simulink model "power_HEV_powertrain"  (Simulink 8.5)
settings: Solver=ode23tb  StartTime=0.0  StopTime=16  MaxStep=Ts  RelTol=1e-3
InitFcn:
  | Pbatt = 21e3;
  | Vbatt = 100;
  | 
  | Ts = 6e-5;   % time step
  | Kb = -2.6;     % planetary gear ratio
  | 
  | MotorNomSpeed = 1200; %rpm
  | MotorMaxTorque = 400; % Nm
  | AccelGain = 1.1;
undefined symbols (not defined in the file): Hydride, magnitude, Metal, Nickel, speed
libraries: powerlib x47, driveline x32, simulink x11, simulink_extras x9, powerlib_extras x4, electricdrivelib x3, DC6DriveInternalModels x1
(part 1 of 3)
Description:
  | Copyright 2008-2011 The MathWorks, Inc.
CloseFcn:
  | rtwprivate ssgensfun ModelCloseRequest power_HEV_powertrain
settings Model: Creator=MathWorks  LastModifiedBy=Elena  CovSFcnEnable=off  ExtModeAutoUpdateStatusClock=off
settings OptimizationCC: OptimizeBlockIOStorage=off  BufferReuse=off  GlobalBufferReuse=off  ExpressionFolding=off  LocalBlockOutputs=off  InitFltsAndDblsToZero=on
settings DebuggingCC: SignalResolutionControl=TryResolveAllWithWarning  SolverPrmCheckMsg=warning  MultiTaskDSMMsg=warning  MultiTaskCondExecSysMsg=none  SigSpecEnsureSampleTimeMsg=none  FcnCallInpInsideContextMsg=UseLocalSettings  UnknownTsInhSupMsg=none
settings HardwareCC: TargetEndianess=LittleEndian  TargetHWDeviceType=MATLAB Host  ProdEqTarget=off

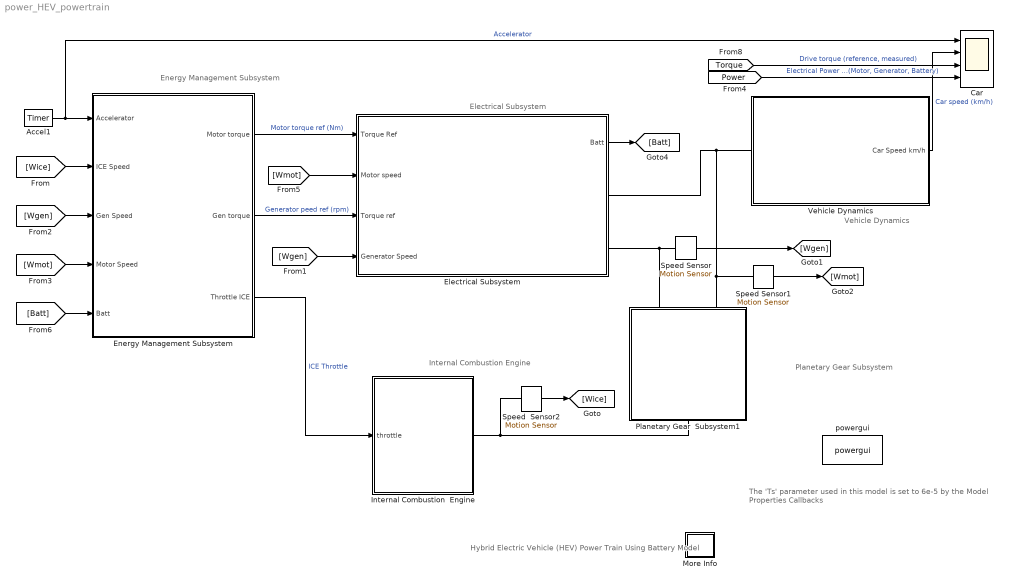
== system power_HEV_powertrain ==
  note: The 'Ts' parameter used in this model
      | is set to 6e-5  by the Model Properties Callbacks
  note: Energy Management
      | Subsystem
  note: Internal Combustion
      | Engine
  note: Planetary Gear
      | Subsystem
  note: Vehicle Dynamics
  note: Hybrid Electric Vehicle (HEV) Power Train Using Battery Model
  note: Electrical Subsystem
  Accel1 : powerlib_extras/Control  Blocks/Timer  t=[0 4 8 13]  e=[0.7 0.1 0.85 -0.7]
  Car : Scope  NumInputPorts=4
      settings: TimeRange=16  YMin=-0.7~-5~-250~-25000  YMax=0.9~75~350~50000  SaveName=ScopeData3  Decimation=10
  Electrical Subsystem : Subsystem
      mask Display: image(imread('power_HEV_powertrain_electrical2.png'))
  Energy Management Subsystem : Subsystem
      mask init:
      | [X1,X1m,X2,X2m,X3,X4,Y1,Y1m,Y2,Y2m,Y3,Y4,color1,color2]=spsdrivelogo;
      | power_max = 57000;
      | speed_at_power_max = 5000;
      | speed_max = 6000;
      | [speed,power,torque,p] = drive_enginemodel('MaskGasoline');
      mask Display:
      | patch([X1 X1m],[Y1 Y1m],color1);
      | patch(X3,Y3,color2);
      | plot([X1 X1m X2 X2m X3 X4],[Y1 Y1m Y2 Y2m Y3 Y4]);
  Internal Combustion  Engine : Subsystem
      mask Display: image(imread('power_HEV_powertrain_THS.jpg'))
  More Info : Subsystem
      settings: OpenFcn=showdemo('power_HEV_powertrain');
      mask Display: disp('?')
  Planetary Gear  Subsystem1 : Subsystem
      mask Display: image(imread('power_HEV_powertrain_planetary2.jpg'));
  Speed Sensor : driveline/Sensors & Actuators/Motion Sensor  Angle=off  x0=0  Velocity=on  Acceleration=off
  Speed Sensor1 : driveline/Sensors & Actuators/Motion Sensor  Angle=off  x0=0  Velocity=on  Acceleration=off
  Speed  Sensor2 : driveline/Sensors & Actuators/Motion Sensor  Angle=off  x0=0  Velocity=on  Acceleration=off
  Vehicle Dynamics : Subsystem
      mask Display: image(imread('power_powertrain_car.jpg'))
  powergui : powerlib/powergui  SimulationMode=Discrete  SolverType=Tustin  SampleTime=6e-5  frequency=60  SPID=off  DisableSnubberDevices=off  DisableRonSwitches=off  DisableVfSwitches=off  SwTol=0  DisplayEquations=off  Interpol=off  methode=off  Ts=0  FunctionMessages=off  echomessages=off  HookPort=off  EnableUseOfTLC=off  x0status=blocks  frequencyindice=0  Pbase=100e6  ErrMax=1e-4  Iterations=50  UnitsV=kV  UnitsW=MW  buscounter=0  RestoreLinks=warning  ResistiveCurrentMeasurement=off  Frange=[0:2:500]  Ylog=off  Xlog=on  ShowGrid=off  save=off  variable=ZData  structure=0  ZoomFFT=on  StartTime=0.0  cycles=1  DisplayStyle=1  fundamental=60  FreqAxis=off  MaxFrequency=1000  frequencyindicesteady=1  RmsSteady=1  display=off
  wires:
  Energy Management Subsystem/1(Motor torque) -> Electrical Subsystem/1(Torque Ref)  "Motor torque ref (Nm)"
  Energy Management Subsystem/2(Gen torque) -> Electrical Subsystem/3(Torque ref)  "Generator peed ref (rpm)"
  Accel1/1 -> Energy Management Subsystem/1(Accelerator), Car/1  "Accelerator"
  Speed Sensor/1 -> [Wgen]
  [Wgen] -> Electrical Subsystem/4(Generator Speed)
  [Wgen] -> Energy Management Subsystem/3(Gen Speed)
  Speed Sensor1/1 -> [Wmot]
  [Wmot] -> Energy Management Subsystem/4(Motor Speed)
  [Wmot] -> Electrical Subsystem/2(Motor speed)
  [Wice] -> Energy Management Subsystem/2(ICE Speed)
  Electrical Subsystem/1(Batt) -> [Batt]
  [Batt] -> Energy Management Subsystem/5(Batt)
  Energy Management Subsystem/3(Throttle ICE) -> Internal Combustion  Engine/1(throttle)  "ICE Throttle"
  Speed  Sensor2/1 -> [Wice]
  [Power] -> Car/4  "Electrical Power (Motor, Generator, Battery)"
  [Torque] -> Car/3  "Drive torque (reference, measured)"
  Vehicle Dynamics/1(Car Speed km/h) -> Car/2  "Car speed (km/h)"
  connections:
  Electrical Subsystem/RConn2 -- Planetary Gear  Subsystem1/RConn1 -- Speed Sensor/LConn1
  Internal Combustion  Engine/RConn1 -- Planetary Gear  Subsystem1/LConn1 -- Speed  Sensor2/LConn1
  Planetary Gear  Subsystem1/RConn2 -- Electrical Subsystem/RConn1 -- Vehicle Dynamics/LConn1 -- Speed Sensor1/LConn1

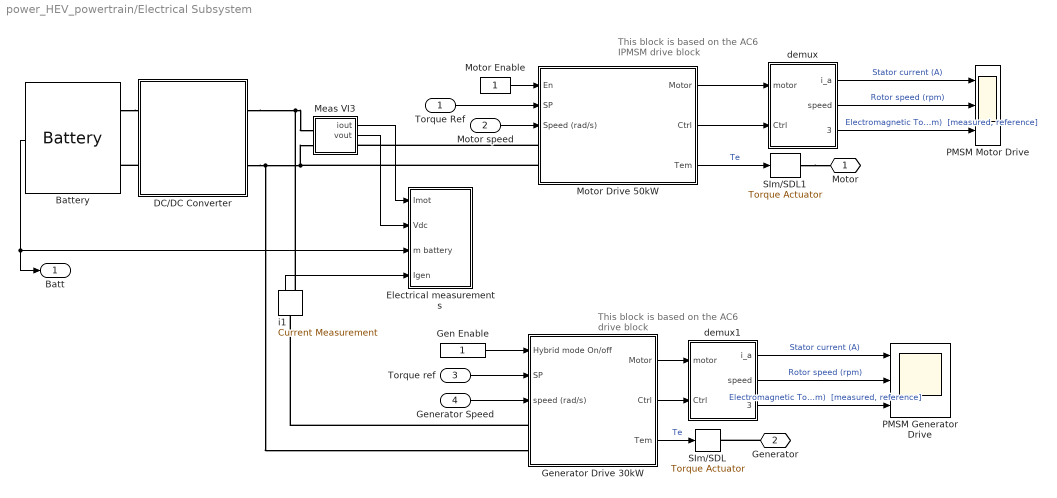
== system power_HEV_powertrain/Electrical Subsystem ==
  note: This block is based on the
      | AC6 IPMSM drive block
  note: This block is based on the AC6
      | drive block
  Torque Ref : Inport
  Motor speed : Inport  Port=2
  Torque ref : Inport  Port=3
  Generator Speed : Inport  Port=4
  Battery : electricdrivelib/Extra Sources/Battery  BatType=Nickel-Metal-Hydride  ShowDetailedParameters=off  NomV=200  NomQ=6.5  SOC=41.53  PresetModel=on  MaxQ=7  FullV=235.5932  Dis_rate=1.3  R=0.30769  Normal_OP=6.25  expZone="[216.9492           1.3]"  current=[50 100]  Units=Time  Batt_Tr=30
  DC/DC Converter : Subsystem
      mask init:
      | [X1,X1m,X2,X2m,X3,X4,Y1,Y1m,Y2,Y2m,Y3,Y4,color1,color2]=spsdrivelogo;
      mask Display:
      | patch([X1 X1m],[Y1 Y1m],color1);
      | patch(X3,Y3,color2);
      | plot([X1 X1m X2 X2m X3 X4],[Y1 Y1m Y2 Y2m Y3 Y4]);
  Electrical measurements : Subsystem
  Gen Enable : Constant
  Generator Drive 30kW : Subsystem
      mask Display: image(imread('power_HEV_powertrain_syncgenerator.jpg'))
  Meas VI3 : Subsystem
  Motor Drive 50kW : Subsystem
      mask Display: image(imread('power_HEV_powertrain_syncmotor.jpg'))
  Motor Enable : Constant
  PMSM Generator Drive : Scope  NumInputPorts=3
      settings: TimeRange=16  YMin=-150~-2000~-35  YMax=150~14000~5  SaveName=simout2  Decimation=10
  PMSM Motor Drive : Scope  NumInputPorts=3
      settings: TimeRange=16  YMin=-250~0~-100  YMax=250~3500~300  SaveName=simout5  Decimation=10
  SIm/SDL : driveline/Sensors & Actuators/Torque Actuator
  SIm/SDL1 : driveline/Sensors & Actuators/Torque Actuator
  demux : Subsystem
  demux1 : Subsystem
  i1 : powerlib/Measurements/Current Measurement  PhasorSimulation=off  OutputType=Complex  PSBequivalent=0
  Motor : PMIOPort  Port=1  Side=Right
  Generator : PMIOPort  Port=2  Side=Right
  Batt : Outport
  wires:
  i1/1 -> Electrical measurements/4(Igen)
  Meas VI3/2(vout) -> Electrical measurements/2(Vdc)
  Meas VI3/1(iout) -> Electrical measurements/1(Imot)
  Torque ref/1 -> Generator Drive 30kW/2(SP)
  Generator Speed/1 -> Generator Drive 30kW/3(speed (rad/s))
  Gen Enable/1 -> Generator Drive 30kW/1(Hybrid mode On/off)
  Battery/1 -> Electrical measurements/3(m battery), Batt/1
  Generator Drive 30kW/3(Tem) -> SIm/SDL/1  "Te"
  demux1/2(speed) -> PMSM Generator Drive/2  "Rotor speed (rpm)"
  demux1/3(Torque) -> PMSM Generator Drive/3  "Electromagnetic Torque (Nm)  [measured, reference]"
  demux1/1(i_a) -> PMSM Generator Drive/1  "Stator current (A)"
  Generator Drive 30kW/1(Motor) -> demux1/1(motor)
  Generator Drive 30kW/2(Ctrl) -> demux1/2(Ctrl)
  Motor Enable/1 -> Motor Drive 50kW/1(En)
  Motor speed/1 -> Motor Drive 50kW/3(Speed (rad/s))
  Torque Ref/1 -> Motor Drive 50kW/2(SP)
  Motor Drive 50kW/3(Tem) -> SIm/SDL1/1  "Te"
  Motor Drive 50kW/1(Motor) -> demux/1(motor)
  Motor Drive 50kW/2(Ctrl) -> demux/2(Ctrl)
  demux/2(speed) -> PMSM Motor Drive/2  "Rotor speed (rpm)"
  demux/3(Torque) -> PMSM Motor Drive/3  "Electromagnetic Torque (Nm)  [measured, reference]"
  demux/1(i_a) -> PMSM Motor Drive/1  "Stator current (A)"
  connections:
  DC/DC Converter/LConn2 -- Battery/LConn2
  Battery/LConn1 -- DC/DC Converter/LConn1
  Generator/RConn1 -- SIm/SDL/RConn1
  Motor Drive 50kW/LConn1 -- Meas VI3/RConn1
  DC/DC Converter/RConn1 -- Meas VI3/LConn1 -- i1/RConn1
  Generator Drive 30kW/LConn1 -- i1/LConn1
  DC/DC Converter/RConn2 -- Generator Drive 30kW/LConn2 -- Motor Drive 50kW/LConn2 -- Meas VI3/LConn2
  SIm/SDL1/RConn1 -- Motor/RConn1

== system power_HEV_powertrain/Energy Management Subsystem ==
  Accelerator : Inport
  ICE Speed : Inport  Port=2
  Gen Speed : Inport  Port=3
  Motor Speed : Inport  Port=4
  Batt : Inport  Port=5
  " 2" : Gain  Gain=-1
  Battery Management System : Subsystem
      mask init:
      | [X1,X1m,X2,X2m,X3,X4,Y1,Y1m,Y2,Y2m,Y3,Y4,color1,color2]=spsdrivelogo;
      mask Display:
      | patch([X1 X1m],[Y1 Y1m],color1);
      | patch(X3,Y3,color2);
      | plot([X1 X1m X2 X2m X3 X4],[Y1 Y1m Y2 Y2m Y3 Y4]);
  Drive torque1 : Product  Inputs=**  OutDataTypeStr=double
  Hybrid Management System : Subsystem
      mask init:
      | [X1,X1m,X2,X2m,X3,X4,Y1,Y1m,Y2,Y2m,Y3,Y4,color1,color2]=spsdrivelogo;
      mask Display:
      | patch([X1 X1m],[Y1 Y1m],color1);
      | patch(X3,Y3,color2);
      | plot([X1 X1m X2 X2m X3 X4],[Y1 Y1m Y2 Y2m Y3 Y4]);
  ICE Speed Controller : Subsystem  mask(Speed controller){SwK=Speed regulation, bs=1800, ramp=[-5000,5000]*10, kp=0.01, ki=0.1, fc=100, ctrl_sat=[0,1], Tsc=Ts}
      mask prompts: SwK "Regulation type"; bs "Base speed (rpm)"; ramp "Speed reference ramp (rpm/s) [deceleration,acceleration]"; kp "Proportional gain"; ki "Integral gain"; fc "Speed measurement - low-pass filter cutoff frequency (Hz)"; ctrl_sat "Controller output torque saturation (N.m) [negative,positive]"; Tsc "Controller sampling time (s)"
      mask help: This block implements a PI speed regulator.
      mask init:
      | [X1,X1m,X2,X2m,X3,X4,Y1,Y1m,Y2,Y2m,Y3,Y4,color1,color2]=spsdrivelogo;
      mask TypeOptions SwK: Speed regulation | Torque regulation
      mask Display:
      | patch([X1 X1m],[Y1 Y1m],color1);
      | patch(X3,Y3,color2);
      | plot([X1 X1m X2 X2m X3 X4],[Y1 Y1m Y2 Y2m Y3 Y4]);
  Rate Limiter : RateLimiter  RisingSlewLimit=10  FallingSlewLimit=-10  SampleTimeMode=inherited
  Scope2 : Scope  NumInputPorts=2
      settings: TimeRange=10  YMin=0~0  YMax=525~7500  SaveName=ScopeData13  Decimation=10
  Terminator : Terminator
  Torque limitation : Subsystem
      mask Display: plot([0;1800;2000;2500;3000;3500], [1;1;0.90*1;0.72*1;0.6*1;0.51*1])
  Motor torque : Outport
  Gen torque : Outport  Port=2
  Throttle ICE : Outport  Port=3
  wires:
  Gen Speed/1 -> Hybrid Management System/6(Generator speed (rad/s))  "Generator speed (rad/s)"
  Motor Speed/1 -> Hybrid Management System/5(Motor speed (rad/s)), Drive torque1/2, Torque limitation/2(N rad/s)  "Motor speed (rad/s)"
  Batt/1 -> Battery Management System/1(Batt)
  Accelerator/1 -> Rate Limiter/1
  ICE Speed/1 -> Hybrid Management System/7(ICE speed (rad/s)), ICE Speed Controller/3(N)
  Hybrid Management System/3(Hybrid Enable) -> ICE Speed Controller/1(En)
  Hybrid Management System/1(Motor torque ref) -> Motor torque/1
  Hybrid Management System/2(Gen torque ref) -> " 2"/1
  ICE Speed Controller/1(Torque*) -> Throttle ICE/1
  ICE Speed Controller/2(Ctrl) -> Terminator/1
  Torque limitation/1(torque) -> Drive torque1/1, Hybrid Management System/3(Drive torque), Scope2/1  "Required torque"
  Drive torque1/1 -> Scope2/2, Hybrid Management System/4(Drive power)  "Required drive power"
  Hybrid Management System/4(ICE speed ref (rpm)) -> ICE Speed Controller/2(N*)
  Battery Management System/1(Battery power) -> Hybrid Management System/1(Recharge power)
  Battery Management System/2(Battery limit) -> Hybrid Management System/2(Battery Limit)
  Rate Limiter/1 -> Torque limitation/1(Torque)
  " 2"/1 -> Gen torque/1

== system power_HEV_powertrain/Internal Combustion  Engine ==
  throttle : Inport
  Driveline Environment : driveline/Solver & Inertias/Driveline Environment  PortType=p1  BlockClass=Solver  PhysicalDomain=driveline_domain  SimulationMode=Dynamics  ModeIteration=off  DefaultClutchVelocityTolerance=1e-3  DefaultUseAutoClutchVelocityTolerance=on
  Gasoline Engine : driveline/Vehicle Components/Gasoline Engine  power_max=57000+57000  speed_at_power_max=5000  speed_max=6000
  Housing : driveline/Solver & Inertias/Housing
  ICE : Scope  NumInputPorts=4
      settings: TimeRange=16  YMin=0~0~-10~-5000  YMax=1~5500~130~50000  SaveName=ScopeData7  Decimation=10
  ICE friction 57 kW @ 5000 rpm : driveline/Dynamic Elements/Torsional  Spring-Damper  k=0  c=0.2079  x0=0  Backlash=0
  Inertia : driveline/Solver & Inertias/Inertia  PortType=p1  BlockClass=Inertia  PhysicalDomain=driveline_domain  I=0.25  Ip=[]  Iv=[]  ShowLeft=off  ShowRight=on
  Motion Sensor : driveline/Sensors & Actuators/Motion Sensor  Angle=off  x0=0  Velocity=on  Acceleration=off
  Product : Product  RndMeth=Zero
  Product1 : Product  RndMeth=Zero
  T1 : driveline/Sensors & Actuators/Torque Sensor
  rad/s to rpm : Constant  Value=60/(2*pi)
  Engine : PMIOPort  Port=1  Side=Right
  tag scope: T_ICE=global
  wires:
  rad/s to rpm/1 -> Product/2
  Motion Sensor/1 -> Product/1, Product1/1
  throttle/1 -> ICE/1, Gasoline Engine/1  "Throttle"
  Product/1 -> ICE/2  "Engine speed (rpm)"
  Product1/1 -> ICE/4  "engine power (w)"
  T1/1 -> Product1/2, [T_ICE], ICE/3  "engine torque (Nm)"
  connections:
  ICE friction 57 kW @ 5000 rpm/LConn1 -- T1/LConn1 -- Inertia/RConn1 -- Motion Sensor/LConn1 -- Gasoline Engine/RConn1 -- Driveline Environment/LConn1
  T1/RConn1 -- Engine/RConn1
  Housing/RConn1 -- ICE friction 57 kW @ 5000 rpm/RConn1

== system power_HEV_powertrain/More Info ==

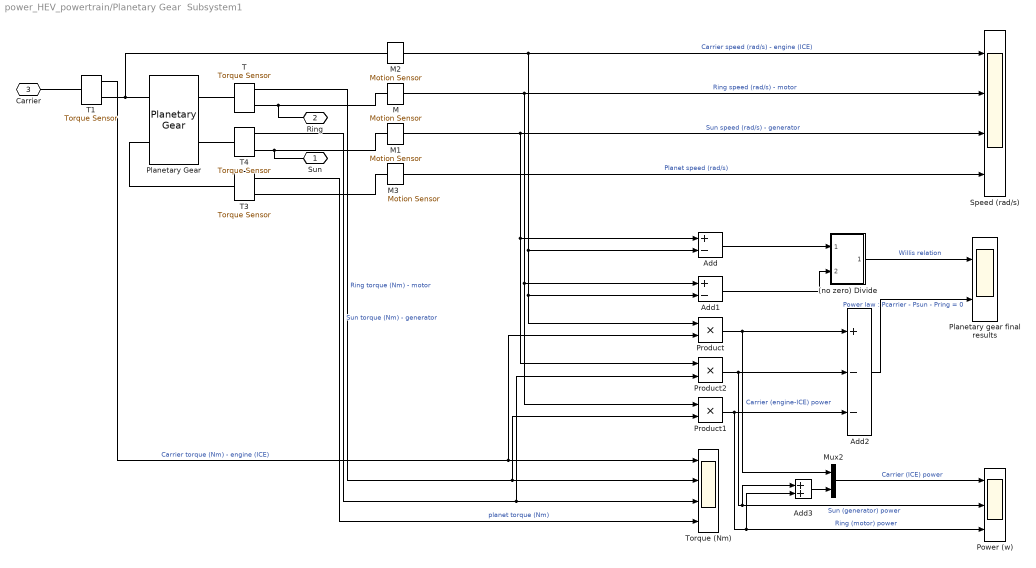
== system power_HEV_powertrain/Planetary Gear  Subsystem1 ==
  (no zero) Divide : Subsystem
  Add : Sum  Inputs=+-
  Add1 : Sum  Inputs=+-
  Add2 : Sum  Inputs=+--
  Add3 : Sum
  M{,1..3} (4 alike) : driveline/Sensors & Actuators/Motion Sensor  Angle=off  x0=0  Velocity=on  Acceleration=off
  Mux2 : Mux  Inputs=2
  Planetary Gear : driveline/Gears/Planetary Gear  Ratio=-Kb  Show=on  LinearizationFlag=off  ValidatorFcn=drive_planetarygearblock
  Planetary gear final results : Scope  NumInputPorts=2
      settings: TimeRange=16  YMin=-3~-1e-010  YMax=0~3e-010  Decimation=10
  Power (w) : Scope  NumInputPorts=3
      settings: TimeRange=16  YMin=-10000~-10000~-2000  YMax=60000~50000~12000  Decimation=10
  Product : Product  RndMeth=Zero
  Product1 : Product  RndMeth=Zero
  Product2 : Product  RndMeth=Zero
  Speed (rad/s) : Scope  NumInputPorts=4
      settings: TimeRange=16  YMin=-100~-20~-200~-400  YMax=500~120~1200~100  SaveName=ScopeData2  Decimation=10
  T{,1,3..4} (4 alike) : driveline/Sensors & Actuators/Torque Sensor
  Torque (Nm) : Scope  NumInputPorts=4
      settings: TimeRange=16  YMin=-50~-20~-10~-2e-013  YMax=150~100~40~6.000000000000001e-013  SaveName=ScopeData4  Decimation=10
  Sun : PMIOPort  Port=1  Side=Right
  Ring : PMIOPort  Port=2  Side=Right
  Carrier : PMIOPort  Port=3  Side=Left
  wires:
  M/1 -> Add1/1, Product1/1, Speed (rad/s)/2  "Ring speed (rad/s) - motor"
  M1/1 -> Speed (rad/s)/3, Add/1, Product2/1  "Sun speed (rad/s) - generator"
  T/1 -> Torque (Nm)/2, Product1/2  "Ring torque (Nm) - motor"
  M2/1 -> Speed (rad/s)/1, Add/2, Add1/2, Product/1  "Carrier speed (rad/s) - engine (ICE)"
  M3/1 -> Speed (rad/s)/4  "Planet speed (rad/s)"
  T3/1 -> Torque (Nm)/4  "planet torque (Nm)"
  T4/1 -> Torque (Nm)/3, Product2/2  "Sun torque (Nm) - generator"
  Add1/1 -> (no zero) Divide/2(SP2)
  (no zero) Divide/1(WR) -> Planetary gear final results/1  "Willis relation"
  Product/1 -> Add2/1, Mux2/1  "Carrier (engine-ICE) power"
  Product2/1 -> Add2/2, Power (w)/2, Add3/1  "Sun (generator) power"
  Product1/1 -> Add2/3, Power (w)/3, Add3/2  "Ring (motor) power"
  Add2/1 -> Planetary gear final results/2  "Power law : Pcarrier - Psun - Pring = 0"
  T1/1 -> Torque (Nm)/1, Product/2  "Carrier torque (Nm) - engine (ICE)"
  Add3/1 -> Mux2/2
  Mux2/1 -> Power (w)/1  "Carrier (ICE) power"
  Add/1 -> (no zero) Divide/1(SP1)
  connections:
  Planetary Gear/LConn1 -- M2/LConn1 -- T1/RConn1
  M1/LConn1 -- T4/RConn1 -- Sun/RConn1
  Planetary Gear/RConn1 -- T/LConn1
  Planetary Gear/RConn2 -- T4/LConn1
  T3/LConn1 -- Planetary Gear/LConn2
  M/LConn1 -- T/RConn1 -- Ring/RConn1
  T3/RConn1 -- M3/LConn1
  T1/LConn1 -- Carrier/RConn1

== system power_HEV_powertrain/Vehicle Dynamics ==
  Differential : driveline/Gears/Differential  R=1  ValidatorFcn=drive_differentialgearblock  SimDrivelineLibraryVersion=1.1
  Housing : driveline/Solver & Inertias/Housing
  Longitudinal Vehicle Dynamics : driveline/Vehicle Components/Longitudinal Vehicle Dynamics  m=1325  a=1.35  b=1.35  h=0.5  FA=2.57  C_d=0.26  v0=0
  Simple Gear : driveline/Gears/Simple Gear  PortType=p1  BlockClass=SimpleGear  PhysicalDomain=driveline_domain  Reversing=off  Ratio=4.113
  Terminator : Terminator
  Terminator1 : Terminator
  Tire : driveline/Vehicle Components/Tire  r_e=0.3  F_z=3000  F_x_max=3500  kappa_max=10  sigma_k=0.2
  Tire1 : driveline/Vehicle Components/Tire  r_e=0.3  F_z=3000  F_x_max=3500  kappa_max=10  sigma_k=0.2
  Torque after gear1 : driveline/Sensors & Actuators/Torque Sensor
  Total friction : driveline/Dynamic Elements/Torsional  Spring-Damper  k=0  c=0.1  x0=0  Backlash=0
  Transmision inertia : driveline/Solver & Inertias/Inertia  PortType=p1  BlockClass=Inertia  PhysicalDomain=driveline_domain  I=0.5  Ip=[]  Iv=[]  ShowLeft=off  ShowRight=on
  m/s to km/h : Gain  Gain=(60*60)/1000
  road angle : Constant  Value=0
  tire inertia : driveline/Solver & Inertias/Inertia  PortType=p1  BlockClass=Inertia  PhysicalDomain=driveline_domain  I=0.5  Ip=[]  Iv=[]  ShowLeft=off  ShowRight=on
  tire inertia1 : driveline/Solver & Inertias/Inertia  PortType=p1  BlockClass=Inertia  PhysicalDomain=driveline_domain  I=0.5  Ip=[]  Iv=[]  ShowLeft=off  ShowRight=on
  Drive Shaft : PMIOPort  Port=1  Side=Left
  Car Speed km/h : Outport
  tag scope: DriveTorque=global
  wires:
  road angle/1 -> Longitudinal Vehicle Dynamics/3
  Tire1/2 -> Longitudinal Vehicle Dynamics/1
  Tire/2 -> Longitudinal Vehicle Dynamics/2
  Tire1/1 -> Terminator/1
  Tire/1 -> Terminator1/1
  Longitudinal Vehicle Dynamics/1 -> Tire/1, Tire1/1, m/s to km/h/1
  Longitudinal Vehicle Dynamics/2 -> Tire1/2
  Longitudinal Vehicle Dynamics/3 -> Tire/2
  m/s to km/h/1 -> Car Speed km/h/1
  Torque after gear1/1 -> [DriveTorque]  "Drive shaft torque"
  connections:
  Differential/RConn1 -- Tire1/LConn1 -- tire inertia1/RConn1
  Differential/RConn2 -- Tire/LConn1 -- tire inertia/RConn1
  Drive Shaft/RConn1 -- Torque after gear1/LConn1
  Torque after gear1/RConn1 -- Simple Gear/LConn1 -- Total friction/RConn1
  Differential/LConn1 -- Simple Gear/RConn1 -- Transmision inertia/RConn1
  Housing/RConn1 -- Total friction/LConn1

== system power_HEV_powertrain/Electrical Subsystem/DC/DC Converter ==
  Bus DC controller : Subsystem
  DC/DC converter : Subsystem
  Ubus Ref : Constant  Value=500
  +Vdc Bus : PMIOPort  Tag=PMCPort  Port=1  Side=Right
  -Vdc Bus : PMIOPort  Tag=PMCPort  Port=2  Side=Right
  + battery : PMIOPort  Tag=PMCPort  Port=3  Side=Left
  - battery : PMIOPort  Tag=PMCPort  Port=4  Side=Left
  wires:
  Ubus Ref/1 -> Bus DC controller/2(Uref)
  Bus DC controller/1(Duty cycle) -> DC/DC converter/1(Duty Cycle)
  DC/DC converter/1(UBus) -> Bus DC controller/1(Ubus)
  connections:
  +Vdc Bus/RConn1 -- DC/DC converter/LConn1
  -Vdc Bus/RConn1 -- DC/DC converter/LConn2
  + battery/RConn1 -- DC/DC converter/RConn1
  - battery/RConn1 -- DC/DC converter/RConn2

== system power_HEV_powertrain/Electrical Subsystem/Electrical measurements ==
  Imot : Inport
  Vdc : Inport  Port=2
  m battery : Inport  Port=3
  Igen : Inport  Port=4
  Bus Selector : BusSelector  OutputSignals=Voltage (V),Current (A),SOC (%)
  Electricals : Scope  NumInputPorts=4
      settings: TimeRange=16  YMin=420~100~-100~39.5  YMax=520~600~150~42.5  SaveName=simout1  Decimation=10
  Mux : Mux  Inputs=2
  Mux1 : Mux  Inputs=3
  Mux2 : Mux  Inputs=3
  Product1 : Product  RndMeth=Zero
  Product2 : Product  RndMeth=Zero
  Product3 : Product  RndMeth=Zero
  tag scope: Power=global
  wires:
  Product2/1 -> Mux1/1  "Motor Power (W)"
  Product1/1 -> Mux1/2  "Generator power (W)"
  Product3/1 -> Mux1/3  "Battery power (W)"
  Imot/1 -> Product2/1, Mux2/1
  Mux1/1 -> [Power]
  m battery/1 -> Bus Selector/1
  Bus Selector/1 -> Mux/2, Product3/1  "<Voltage (V)>"
  Bus Selector/2 -> Product3/2, Mux2/2  "<Current (A)>"
  [V_DCDC] -> Electricals/1  "DC/DC converter Voltage (Reference, Measured)"
  Mux/1 -> Electricals/2  "Voltage (DC bus, Battery)"
  Mux2/1 -> Electricals/3  "Current (Motor, Battery, Generator)"
  Igen/1 -> Product1/1, Mux2/3
  Bus Selector/3 -> Electricals/4  "<SOC (%)>"
  Vdc/1 -> Product2/2, Product1/2, Mux/1

== system power_HEV_powertrain/Electrical Subsystem/Generator Drive 30kW ==
  Hybrid mode On/off : Inport
  SP : Inport  Port=2
  speed (rad/s) : Inport  Port=3
  Bus Selector : BusSelector  OutputSignals=Rotor speed wm (rad/s),Rotor angle thetam (rad),Electromagnetic torque Te (N*m)
  Measures : electricdrivelib/AC drives/PM Synchronous Motor Drive/Measures
  Mux : Subsystem
  PMSM1 : powerlib/Machines/Permanent Magnet Synchronous Machine  NbPhases=3  FluxDistribution=Sinusoidal  RotorType=Salient-pole  MechanicalLoad=Speed w  PresetModel=No  ShowDetailedParameters=on  MeasurementBus=off  Resistance=0.05  Inductance=0  dqInductances=[0.000635 0.000635]  La=0.000835  MachineConstant=Flux linkage established by magnets (V.s)  Flux=0.192  VoltageCst=34.8249  TorqueCst=0.288  Flat=0  Mechanical=[0.011 0.001889/4 4/4]  PolePairs=1  InitialConditions=[0,0, 0,0,0]  InitialConditions5ph=[0 0 0 0 0 0]  TsPowergui=0  TsBlock=-1  RefAngle=90 degrees behind phase A axis (modified Park)
      settings: AttributesFormatString=\n
  Speed Controller : Subsystem  mask(Speed controller){SwK=Torque regulation, bs=1800, ramp=[-5000,5000], kp=(1/5)/4, ki=(50/5)/4/3, fc=(1000/10)/2, ctrl_sat=[-45,45], Tsc=120e-6}
      mask prompts: SwK "Regulation type"; bs "Base speed (rpm)"; ramp "Speed reference ramp (rpm/s) [deceleration,acceleration]"; kp "Proportional gain"; ki "Integral gain"; fc "Speed measurement - low-pass filter cutoff frequency (Hz)"; ctrl_sat "Controller output torque saturation (N.m) [negative,positive]"; Tsc "Controller sampling time (s)"
      mask help: This block implements a PI speed regulator.
      mask init:
      | [X1,X1m,X2,X2m,X3,X4,Y1,Y1m,Y2,Y2m,Y3,Y4,color1,color2]=spsdrivelogo;
      mask TypeOptions SwK: Speed regulation | Torque regulation
      mask Display:
      | patch([X1 X1m],[Y1 Y1m],color1);
      | patch(X3,Y3,color2);
      | plot([X1 X1m X2 X2m X3 X4],[Y1 Y1m Y2 Y2m Y3 Y4]);
  Three-phase Inverter : Subsystem  mask(SPSdrives Converter){Arms=3, SnubberResistance=5000, SnubberCapacitance=inf, Device=IGBT / Diodes, Ron=1e-3, Lon=0, ForwardVoltages=[0.8,0.8], ForwardVoltage=0, GTOparameters=[0,0], IGBTparameters=[1e-6,2e-6], Measurements=All voltages and currents, SourceFrequency=60, dqInductances=[0.000635,0.000635], Flux=0.192, Resistance=0.05, p=4/4, converterType=Inverter}
      mask prompts: Arms "Number of bridge arms:"; SnubberResistance "Snubber resistance Rs (Ohms)"; SnubberCapacitance "Snubber capacitance Cs (F)"; Device "Power Electronic device"; Ron "Ron (Ohms)"; Lon "Lon (H)"; ForwardVoltages "Forward voltages  [ Device Vf(V) , Diode Vfd(V)]"; ForwardVoltage "Forward voltage Vf (V)"; GTOparameters "[  Tf (s) , Tt (s)  ]"; IGBTparameters "[  Tf (s) , Tt (s)  ]"; SourceFrequency "Source Frequency (Hz)"; dqInductances "PMSM-Inductances [ Ld(H) Lq(H) ]:"; Flux "PMSM-Flux induced by magnets (Wb):"; Resistance "PMSM-Stator resistance Rs (ohm):"; p "PMSM-Pairs of poles p:"; converterType "Converter type:"
      mask init:
      | Ld=dqInductances(1);
      | Lq=dqInductances(2);
      | Fcs=6*SourceFrequency/10;
      settings: OpenFcn=power_openblockproxy();
      mask Help: web(psbhelp);
      mask TypeOptions Arms: 1 | 2 | 3
      mask TypeOptions Device: Diodes | Thyristors | GTO / Diodes | MOSFET / Diodes | IGBT / Diodes | Ideal Switches
      mask TypeOptions Measurements: None | Device voltages | Device currents | UAB UBC UCA UDC voltages | All voltages and currents
      mask TypeOptions converterType: Rectifier | Inverter
      mask Display: plot(0,0,100,100,[39 39 23.8],[71 28 28],[44 56 49.6 56 52.8 56 61 61],[39.2 33.6 32.8 33.6 40.8 33.6 30 12.4],[44 44 44 61 61],[28 71 60 66.4 90],[75 67 83 75 67 83 75 75],[54 42 42 54 54 54 54 66],[61 75 75],[24 24 42],[75 75 61],[66,76,76])
  VECT : Subsystem  mask(VECT){nb_p=4/4, lambda=0.192, freq_max=20e3, Ts_vect=60e-6, h=2}
      mask prompts: nb_p "Motor pairs of poles"; lambda "Flux induced by magnets (Wb)"; freq_max "Maximum switching frequency (Hz)"; Ts_vect "Sampling time (s)"; h "Current hysteresis bandwidth (A)"
      mask help: This block implements a vector controller.
      mask init:
      | [X1,X1m,X2,X2m,X3,X4,Y1,Y1m,Y2,Y2m,Y3,Y4,color1,color2]=spsdrivelogo;
      mask Display:
      | patch([X1 X1m],[Y1 Y1m],color1);
      | patch(X3,Y3,color2);
      | plot([X1 X1m X2 X2m X3 X4],[Y1 Y1m Y2 Y2m Y3 Y4]);
  + : PMIOPort  Port=1  Side=Left
  - : PMIOPort  Port=2  Side=Left
  Motor : Outport
  Ctrl : Outport  Port=2
  Tem : Outport  Port=3
  wires:
  Hybrid mode On/off/1 -> VECT/1(En), Speed Controller/3(En)
  SP/1 -> Speed Controller/2(N*)
  Speed Controller/1(Torque*) -> VECT/2(Torque*)
  Bus Selector/1 -> Speed Controller/1(N)  "<Rotor speed wm (rad/s)>"
  PMSM1/1 -> Mux/2(m), Bus Selector/1, Motor/1
  speed (rad/s)/1 -> PMSM1/1
  Bus Selector/3 -> Tem/1  "<Electromagnetic torque Te (N*m)>"
  Measures/1 -> VECT/4(I_abc)
  Speed Controller/2(Ctrl) -> Ctrl/1
  VECT/1(sig*) -> Mux/1(sig*)
  Mux/1(Ctrl) -> Three-phase Inverter/1(ctrl)
  Bus Selector/2 -> VECT/3(teta)  "<Rotor angle thetam (rad)>"
  connections:
  -/RConn1 -- Three-phase Inverter/RConn2
  +/RConn1 -- Three-phase Inverter/RConn1
  Measures/RConn1 -- PMSM1/LConn1
  Measures/RConn2 -- PMSM1/LConn2
  Measures/RConn3 -- PMSM1/LConn3
  Three-phase Inverter/LConn1 -- Measures/LConn1
  Measures/LConn2 -- Three-phase Inverter/LConn2
  Three-phase Inverter/LConn3 -- Measures/LConn3

== system power_HEV_powertrain/Electrical Subsystem/Meas VI3 ==
  V1 : powerlib/Measurements/Voltage Measurement  PhasorSimulation=off  OutputType=Complex  PSBequivalent=0
  i1 : powerlib/Measurements/Current Measurement  PhasorSimulation=off  OutputType=Complex  PSBequivalent=0
  iref : PMIOPort  Port=1  Side=Right
  + : PMIOPort  Tag=PMCPort  Port=2  Side=Left
  vref : PMIOPort  Port=3  Side=Left
  iout : Outport
  vout : Outport  Port=2
  wires:
  V1/1 -> vout/1
  i1/1 -> iout/1
  connections:
  vref/RConn1 -- V1/LConn2
  iref/RConn1 -- i1/RConn1
  i1/LConn1 -- +/RConn1 -- V1/LConn1

== system power_HEV_powertrain/Electrical Subsystem/Motor Drive 50kW ==
  En : Inport
  SP : Inport  Port=2
  Speed (rad/s) : Inport  Port=3
  500 Vdc 50kW PMSM : powerlib/Machines/Permanent Magnet Synchronous Machine  NbPhases=3  FluxDistribution=Sinusoidal  RotorType=Salient-pole  MechanicalLoad=Speed w  PresetModel=No  ShowDetailedParameters=on  MeasurementBus=off  Resistance=0.0065  Inductance=0  dqInductances="[0.001597972349731   0.002057052250467]"  La=0.000835  MachineConstant=Flux linkage established by magnets (V.s)  Flux=0.175666143629361  VoltageCst=127.4493  TorqueCst=1.054  Flat=0  Mechanical=[0.089 0.005 4]  PolePairs=4  InitialConditions=[0,0,0,0]  InitialConditions5ph=[0 0 0 0 0 0]  TsPowergui=0  TsBlock=-1  RefAngle=90 degrees behind phase A axis (modified Park)
      settings: AttributesFormatString=\n
  Bus Selector : BusSelector  OutputSignals=Rotor speed wm (rad/s),Rotor angle thetam (rad),Electromagnetic torque Te (N*m)
  Measures : electricdrivelib/AC drives/PM Synchronous Motor Drive/Measures
  Mux : Subsystem
  Speed Controller : Subsystem  mask(Speed controller){SwK=Torque regulation, bs=3000, ramp=[-10000,10000], kp=1/5, ki=50/5, fc=1000/10, ctrl_sat=[-400,400], Tsc=120e-6}
      mask prompts: SwK "Regulation type"; bs "Base speed (rpm)"; ramp "Speed reference ramp (rpm/s) [deceleration,acceleration]"; kp "Proportional gain"; ki "Integral gain"; fc "Speed measurement - low-pass filter cutoff frequency (Hz)"; ctrl_sat "Controller output torque saturation (N.m) [negative,positive]"; Tsc "Controller sampling time (s)"
      mask help: This block implements a PI speed regulator.
      mask init:
      | [X1,X1m,X2,X2m,X3,X4,Y1,Y1m,Y2,Y2m,Y3,Y4,color1,color2]=spsdrivelogo;
      mask TypeOptions SwK: Speed regulation | Torque regulation
      mask Display:
      | patch([X1 X1m],[Y1 Y1m],color1);
      | patch(X3,Y3,color2);
      | plot([X1 X1m X2 X2m X3 X4],[Y1 Y1m Y2 Y2m Y3 Y4]);
  Three-phase Inverter : Subsystem  mask(SPSdrives Converter){Arms=3, SnubberResistance=5000, SnubberCapacitance=inf, Device=IGBT / Diodes, Ron=1e-3, Lon=0, ForwardVoltages=[0.8,0.8], ForwardVoltage=0, GTOparameters=[0,0], IGBTparameters=[1e-6,2e-6], Measurements=All voltages and currents, SourceFrequency=60, dqInductances=[0.001597972349731   0.002057052250467], Flux=0.175666143629361, Resistance=0.0065, p=4, converterType=Inverter}
      mask prompts: Arms "Number of bridge arms:"; SnubberResistance "Snubber resistance Rs (Ohms)"; SnubberCapacitance "Snubber capacitance Cs (F)"; Device "Power Electronic device"; Ron "Ron (Ohms)"; Lon "Lon (H)"; ForwardVoltages "Forward voltages  [ Device Vf(V) , Diode Vfd(V)]"; ForwardVoltage "Forward voltage Vf (V)"; GTOparameters "[  Tf (s) , Tt (s)  ]"; IGBTparameters "[  Tf (s) , Tt (s)  ]"; SourceFrequency "Source Frequency (Hz)"; dqInductances "PMSM-Inductances [ Ld(H) Lq(H) ]:"; Flux "PMSM-Flux induced by magnets (Wb):"; Resistance "PMSM-Stator resistance Rs (ohm):"; p "PMSM-Pairs of poles p:"; converterType "Converter type:"
      mask init:
      | Ld=dqInductances(1);
      | Lq=dqInductances(2);
      | Fcs=6*SourceFrequency/10;
      settings: OpenFcn=power_openblockproxy();
      mask Help: web(psbhelp);
      mask TypeOptions Arms: 1 | 2 | 3
      mask TypeOptions Device: Diodes | Thyristors | GTO / Diodes | MOSFET / Diodes | IGBT / Diodes | Ideal Switches
      mask TypeOptions Measurements: None | Device voltages | Device currents | UAB UBC UCA UDC voltages | All voltages and currents
      mask TypeOptions converterType: Rectifier | Inverter
      mask Display: plot(0,0,100,100,[39 39 23.8],[71 28 28],[44 56 49.6 56 52.8 56 61 61],[39.2 33.6 32.8 33.6 40.8 33.6 30 12.4],[44 44 44 61 61],[28 71 60 66.4 90],[75 67 83 75 67 83 75 75],[54 42 42 54 54 54 54 66],[61 75 75],[24 24 42],[75 75 61],[66,76,76])
  Torque limitation : Subsystem
      mask Display: plot([0;1800;2000;2500;3000;3500], [1;1;0.90*1;0.72*1;0.6*1;0.51*1])
  VECT controller : Subsystem  mask(VECT){nb_p=4, dqInductances=[0.001597972349731   0.002057052250467], lambda=0.175666143629361, Ts_vect=60e-6}
      mask prompts: nb_p "Motor pairs of poles"; dqInductances "Inductances [ Ld(H) Lq(H) ]:"; lambda "Flux induced by magnets (Wb)"; Ts_vect "Sampling time (s)"
      mask help: This block implements a vector controller.
      mask init:
      | [X1,X1m,X2,X2m,X3,X4,Y1,Y1m,Y2,Y2m,Y3,Y4,color1,color2]=spsdrivelogo;
      | ib = lambda/(dqInductances(2)-dqInductances(1));
      | Teb = 3/2*nb_p*lambda*ib;
      | Ld = dqInductances(1);
      | Lq = dqInductances(2);
      | lam = lambda;
      | p=nb_p;
      | ib = lam/(Lq-Ld);
      | iqn = 0:0.01:3;
      | ten = iqn/2.*(sqrt(4*iqn.*iqn+1)+1);
      mask Display:
      | patch([X1 X1m],[Y1 Y1m],color1);
      | patch(X3,Y3,color2);
      | plot([X1 X1m X2 X2m X3 X4],[Y1 Y1m Y2 Y2m Y3 Y4]);
  + : PMIOPort  Port=1  Side=Left
  - : PMIOPort  Port=2  Side=Left
  Motor : Outport
  Ctrl : Outport  Port=2
  Tem : Outport  Port=3
  wires:
  Mux/1(Ctrl) -> Three-phase Inverter/1(ctrl)
  VECT controller/1(sig*) -> Mux/1(sig*)
  Speed Controller/2(Ctrl) -> Ctrl/1
  Speed (rad/s)/1 -> 500 Vdc 50kW PMSM/1
  500 Vdc 50kW PMSM/1 -> Bus Selector/1, Mux/2(m), Motor/1
  Bus Selector/3 -> Tem/1  "<Electromagnetic torque Te (N*m)>"
  Bus Selector/1 -> VECT controller/3(w), Speed Controller/1(N), Torque limitation/1(N rad/s)  "<Rotor speed wm (rad/s)>"
  En/1 -> Speed Controller/3(En), VECT controller/1(En)
  Speed Controller/1(Torque*) -> VECT controller/2(Torque*)
  Measures/1 -> VECT controller/5(I_abc)
  Bus Selector/2 -> VECT controller/4(teta)  "<Rotor angle thetam (rad)>"
  Torque limitation/1(torque) -> Speed Controller/2(N*)
  SP/1 -> Torque limitation/2(Torque)
  connections:
  Three-phase Inverter/LConn3 -- Measures/LConn3
  Measures/LConn2 -- Three-phase Inverter/LConn2
  Three-phase Inverter/LConn1 -- Measures/LConn1
  Measures/RConn3 -- 500 Vdc 50kW PMSM/LConn3
  Measures/RConn2 -- 500 Vdc 50kW PMSM/LConn2
  Measures/RConn1 -- 500 Vdc 50kW PMSM/LConn1
  +/RConn1 -- Three-phase Inverter/RConn1
  -/RConn1 -- Three-phase Inverter/RConn2

== system power_HEV_powertrain/Electrical Subsystem/demux ==
  motor : Inport
  Ctrl : Inport  Port=2
  "+ -> -1" : Gain  Gain=30/pi
  Bus Selector : BusSelector  OutputSignals=Stator current is_a (A),Rotor speed wm (rad/s),Electromagnetic torque Te (N*m)
  Bus Selector1 : BusSelector  OutputSignals=Torque reference (Nm)
  Mux1 : Mux  Inputs=2
  i_a : Outport
  speed : Outport  Port=2
  Torque : Outport  Port=3
  wires:
  "+ -> -1"/1 -> speed/1
  motor/1 -> Bus Selector/1
  Ctrl/1 -> Bus Selector1/1
  Bus Selector/2 -> "+ -> -1"/1  "<Rotor speed wm (rad/s)>"
  Bus Selector/3 -> Mux1/1  "<Electromagnetic torque Te (N*m)>"
  Bus Selector1/1 -> Mux1/2  "<Torque reference (Nm)>"
  Mux1/1 -> Torque/1
  Bus Selector/1 -> i_a/1  "<Stator current is_a (A)>"

== system power_HEV_powertrain/Electrical Subsystem/demux1 ==
  motor : Inport
  Ctrl : Inport  Port=2
  "+ -> -1" : Gain  Gain=30/pi
  Bus Selector : BusSelector  OutputSignals=Stator current is_a (A),Rotor speed wm (rad/s),Electromagnetic torque Te (N*m)
  Bus Selector1 : BusSelector  OutputSignals=Torque reference (Nm)
  Mux1 : Mux  Inputs=2
  i_a : Outport
  speed : Outport  Port=2
  Torque : Outport  Port=3
  wires:
  Mux1/1 -> Torque/1
  Bus Selector1/1 -> Mux1/2  "<Torque reference (Nm)>"
  Bus Selector/3 -> Mux1/1  "<Electromagnetic torque Te (N*m)>"
  Bus Selector/2 -> "+ -> -1"/1  "<Rotor speed wm (rad/s)>"
  Ctrl/1 -> Bus Selector1/1
  Bus Selector/1 -> i_a/1  "<Stator current is_a (A)>"
  motor/1 -> Bus Selector/1
  "+ -> -1"/1 -> speed/1

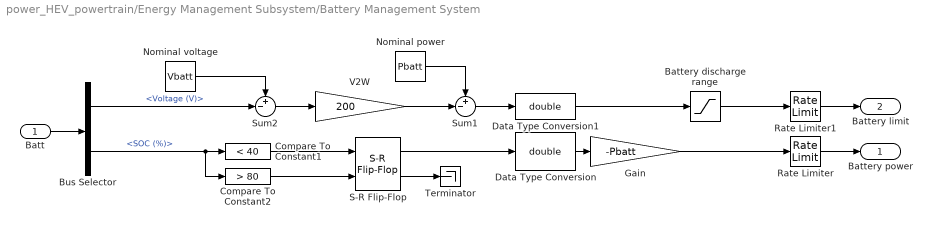
== system power_HEV_powertrain/Energy Management Subsystem/Battery Management System ==
  Batt : Inport
  Battery discharge range : Saturate  UpperLimit=Pbatt  LowerLimit=0
  Bus Selector : BusSelector  OutputSignals=Voltage (V),SOC (%)
  Compare To Constant1 : simulink/Logic and Bit Operations/Compare To Constant  relop=<  const=40  OutDataTypeStr=boolean
  Compare To Constant2 : simulink/Logic and Bit Operations/Compare To Constant  relop=>  const=80  OutDataTypeStr=boolean
  Data Type Conversion : DataTypeConversion  OutDataTypeStr=double  SampleTime=0
  Data Type Conversion1 : DataTypeConversion  OutDataTypeStr=double  SampleTime=0
  Gain : Gain  Gain=-Pbatt
  Nominal power : Constant  Value=Pbatt
  Nominal voltage : Constant  Value=Vbatt
  Rate Limiter : RateLimiter  RisingSlewLimit=Pbatt*2  FallingSlewLimit=-Pbatt*2  SampleTimeMode=inherited
  Rate Limiter1 : RateLimiter  RisingSlewLimit=Pbatt*10  FallingSlewLimit=-Pbatt*10  SampleTimeMode=inherited
  S-R Flip-Flop : simulink_extras/Flip Flops/S-R Flip-Flop  initial_condition=0
  Sum1 : Sum  Inputs=+-|
  Sum2 : Sum  Inputs=+-|
  Terminator : Terminator
  V2W : Gain  Gain=200
  Battery power : Outport
  Battery limit : Outport  Port=2
  wires:
  Batt/1 -> Bus Selector/1
  Gain/1 -> Rate Limiter/1
  S-R Flip-Flop/2 -> Terminator/1
  Bus Selector/2 -> Compare To Constant1/1, Compare To Constant2/1  "<SOC (%)>"
  Data Type Conversion/1 -> Gain/1
  Compare To Constant1/1 -> S-R Flip-Flop/1
  Compare To Constant2/1 -> S-R Flip-Flop/2
  S-R Flip-Flop/1 -> Data Type Conversion/1
  Sum2/1 -> V2W/1
  V2W/1 -> Sum1/2
  Nominal power/1 -> Sum1/1
  Sum1/1 -> Data Type Conversion1/1
  Data Type Conversion1/1 -> Battery discharge range/1
  Battery discharge range/1 -> Rate Limiter1/1
  Bus Selector/1 -> Sum2/2  "<Voltage (V)>"
  Nominal voltage/1 -> Sum2/1
  Rate Limiter1/1 -> Battery limit/1
  Rate Limiter/1 -> Battery power/1

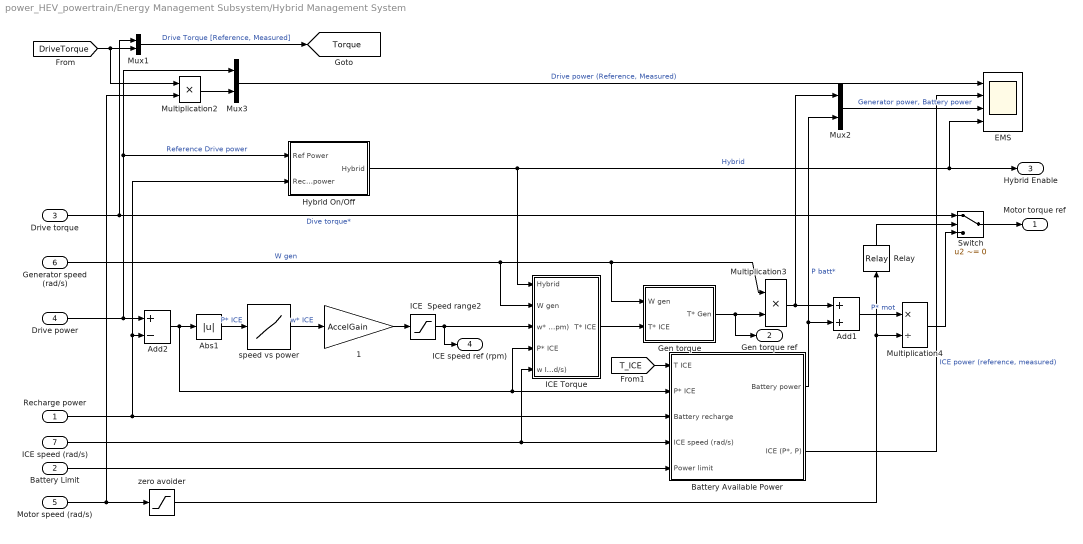
== system power_HEV_powertrain/Energy Management Subsystem/Hybrid Management System ==
  Recharge power : Inport
  Battery Limit : Inport  Port=2
  Drive torque : Inport  Port=3
  Drive power : Inport  Port=4
  Motor speed (rad/s) : Inport  Port=5
  Generator speed (rad/s) : Inport  Port=6
  ICE speed (rad/s) : Inport  Port=7
  " 1" : Gain  Gain=AccelGain
  Abs1 : Abs
  Add1 : Sum
  Add2 : Sum  Inputs=+-
  Battery Available Power : Subsystem
  EMS : Scope  NumInputPorts=4
      settings: TimeRange=16  YMin=-80000~-20000~-30000~0  YMax=80000~100000~30000~1  SaveName=ScopeData5  Decimation=10
  Gen torque : Subsystem
  Hybrid On/Off : Subsystem
  ICE  Speed range2 : Saturate  UpperLimit=5000  LowerLimit=750
  ICE Torque : Subsystem
  Multiplication2 : Product
  Multiplication3 : Product
  Multiplication4 : Product  Inputs=*/
  Mux1 : Mux  Inputs=2
  Mux2 : Mux  Inputs=2
  Mux3 : Mux  Inputs=2
  Relay : Relay  OnSwitchValue=200/30*pi  OffSwitchValue=100/30*pi  OnOutputValue=0  OffOutputValue=1
  Switch : Switch  Criteria=u2 ~= 0
  speed vs power : Lookup  InputValues=power(1:84)  Table=speed(1:84)  SaturateOnIntegerOverflow=on
  zero avoider : Saturate  UpperLimit=inf  LowerLimit=1
  Motor torque ref : Outport
  Gen torque ref : Outport  Port=2
  Hybrid Enable : Outport  Port=3
  ICE speed ref (rpm) : Outport  Port=4
  tag scope: Torque=global
  wires:
  Motor speed (rad/s)/1 -> zero avoider/1, Multiplication2/2
  speed vs power/1 -> " 1"/1  "w* ICE"
  Generator speed (rad/s)/1 -> ICE Torque/2(W gen), Multiplication3/1, Gen torque/1(W gen)  "W gen"
  Multiplication3/1 -> Add1/1, Mux2/1
  Add1/1 -> Multiplication4/1  "P* mot"
  zero avoider/1 -> Relay/1, Multiplication4/2
  Multiplication4/1 -> Switch/3
  Drive torque/1 -> Mux1/1, Switch/1  "Dive torque*"
  Switch/1 -> Motor torque ref/1
  Drive power/1 -> Add2/1, Hybrid On/Off/1(Ref Power), Mux3/1  "Reference Drive power"
  [DriveTorque] -> Mux1/2, Multiplication2/1
  Mux1/1 -> [Torque]  "Drive Torque [Reference, Measured]"
  Abs1/1 -> speed vs power/1  "P* ICE"
  Add2/1 -> Abs1/1, Battery Available Power/2(P* ICE), ICE Torque/4(P* ICE)
  Recharge power/1 -> Battery Available Power/3(Battery recharge), Add2/2, Hybrid On/Off/2(Recharge power)
  ICE speed (rad/s)/1 -> Battery Available Power/4(ICE speed (rad/s)), ICE Torque/5(w ICE (rad/s))
  Battery Available Power/1(Battery power) -> Add1/2, Mux2/2  "P batt*"
  Hybrid On/Off/1(Hybrid) -> ICE Torque/1(Hybrid), EMS/4, Hybrid Enable/1  "Hybrid"
  Relay/1 -> Switch/2
  Battery Limit/1 -> Battery Available Power/5(Power limit)
  Multiplication2/1 -> Mux3/2
  Mux3/1 -> EMS/1  "Drive power (Reference, Measured)"
  Battery Available Power/2("ICE (P*, P)") -> EMS/2  "ICE power (reference, measured)"
  Mux2/1 -> EMS/3  "Generator power, Battery power"
  ICE Torque/1(T* ICE) -> Gen torque/2(T* ICE)
  [T_ICE] -> Battery Available Power/1(T ICE)
  ICE  Speed range2/1 -> ICE speed ref (rpm)/1, ICE Torque/3(w* ICE (rpm))
  " 1"/1 -> ICE  Speed range2/1
  Gen torque/1(T* Gen) -> Multiplication3/2, Gen torque ref/1

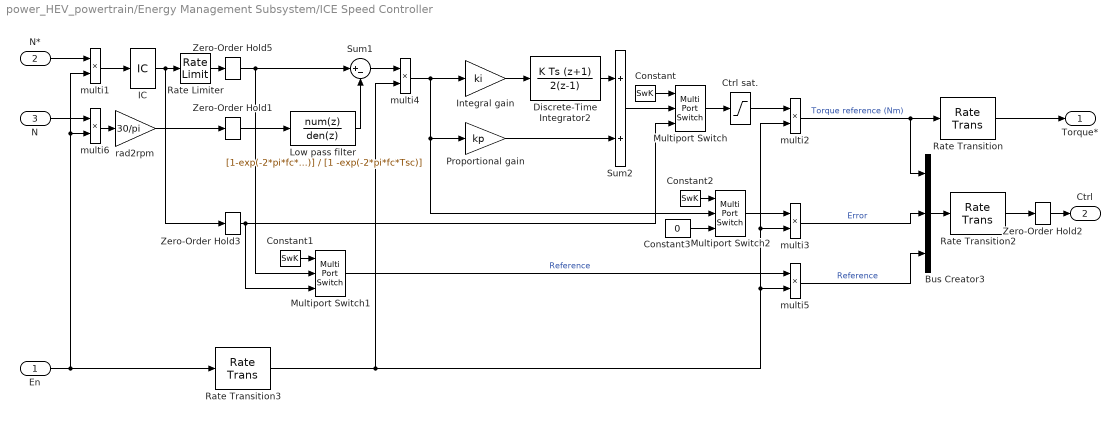
== system power_HEV_powertrain/Energy Management Subsystem/ICE Speed Controller ==
  En : Inport
  N* : Inport  Port=2
  N : Inport  Port=3
  Bus Creator3 : BusCreator  Inputs=3
  Constant : Constant  Value=SwK
  Constant1 : Constant  Value=SwK
  Constant2 : Constant  Value=SwK
  Constant3 : Constant  Value=0
  Ctrl sat. : Saturate  UpperLimit=ctrl_sat(2)  LowerLimit=ctrl_sat(1)
  Discrete-Time Integrator2 : DiscreteIntegrator  IntegratorMethod=Integration: Trapezoidal  SampleTime=Tsc  LimitOutput=on  UpperSaturationLimit=ctrl_sat(2)  LowerSaturationLimit=ctrl_sat(1)
  IC : InitialCondition  Value=0
  Integral gain : Gain  Gain=ki  SaturateOnIntegerOverflow=on  OutDataTypeStr=Inherit: Same as input  ParamDataTypeStr=Inherit: Same as input
  Low pass filter : DiscreteTransferFcn  Numerator=[1-exp(-2*pi*fc*Tsc)]  Denominator=[1 -exp(-2*pi*fc*Tsc)]  SampleTime=Tsc
  Multiport Switch : MultiPortSwitch  Inputs=2  SaturateOnIntegerOverflow=on
  Multiport Switch1 : MultiPortSwitch  Inputs=2  SaturateOnIntegerOverflow=on
  Multiport Switch2 : MultiPortSwitch  Inputs=2  SaturateOnIntegerOverflow=on
  Proportional gain : Gain  Gain=kp  SaturateOnIntegerOverflow=on  OutDataTypeStr=Inherit: Same as input  ParamDataTypeStr=Inherit: Same as input
  Rate Limiter : RateLimiter  RisingSlewLimit=ramp(2)  FallingSlewLimit=ramp(1)  LinearizeAsGain=off
  Rate Transition : RateTransition
  Rate Transition2 : RateTransition
  Rate Transition3 : RateTransition
  Sum1 : Sum  Inputs=|+-  SaturateOnIntegerOverflow=on  InputSameDT=on  OutDataTypeStr=Inherit: Same as first input
  Sum2 : Sum  SaturateOnIntegerOverflow=on  InputSameDT=on  OutDataTypeStr=Inherit: Same as first input
  Zero-Order Hold1 : ZeroOrderHold  SampleTime=Tsc
  Zero-Order Hold2 : ZeroOrderHold  SampleTime=Ts
  Zero-Order Hold3 : ZeroOrderHold  SampleTime=Tsc
  Zero-Order Hold5 : ZeroOrderHold  SampleTime=Tsc
  multi{1..6} (6 alike) : Product
  rad2rpm : Gain  Gain=30/pi  SaturateOnIntegerOverflow=on  OutDataTypeStr=Inherit: Same as input  ParamDataTypeStr=Inherit: Same as input
  Torque* : Outport
  Ctrl : Outport  Port=2
  wires:
  N/1 -> multi6/1
  multi6/1 -> rad2rpm/1
  N*/1 -> multi1/1
  multi1/1 -> IC/1
  Rate Transition3/1 -> multi5/2, multi2/2, multi3/2, multi4/2
  multi4/1 -> Proportional gain/1, Multiport Switch2/2, Integral gain/1
  Low pass filter/1 -> Sum1/2
  multi2/1 -> Bus Creator3/1, Rate Transition/1  "Torque reference (Nm)"
  Multiport Switch1/1 -> multi5/1  "Reference"
  multi5/1 -> Bus Creator3/3  "Reference"
  multi3/1 -> Bus Creator3/2  "Error"
  Multiport Switch2/1 -> multi3/1
  Zero-Order Hold2/1 -> Ctrl/1
  Rate Transition/1 -> Torque*/1
  En/1 -> multi6/2, multi1/2, Rate Transition3/1
  rad2rpm/1 -> Zero-Order Hold1/1
  Constant3/1 -> Multiport Switch2/3
  Constant2/1 -> Multiport Switch2/1
  Zero-Order Hold3/1 -> Multiport Switch1/3, Multiport Switch/3
  Constant1/1 -> Multiport Switch1/1
  Sum2/1 -> Multiport Switch/2
  Constant/1 -> Multiport Switch/1
  Multiport Switch/1 -> Ctrl sat./1
  Zero-Order Hold5/1 -> Multiport Switch1/2, Sum1/1
  Rate Limiter/1 -> Zero-Order Hold5/1
  Bus Creator3/1 -> Rate Transition2/1
  Rate Transition2/1 -> Zero-Order Hold2/1
  Zero-Order Hold1/1 -> Low pass filter/1
  IC/1 -> Zero-Order Hold3/1, Rate Limiter/1
  Proportional gain/1 -> Sum2/2
  Discrete-Time Integrator2/1 -> Sum2/1
  Sum1/1 -> multi4/1
  Integral gain/1 -> Discrete-Time Integrator2/1
  Ctrl sat./1 -> multi2/1

== system power_HEV_powertrain/Energy Management Subsystem/Torque limitation ==
  Torque : Inport
  N rad/s : Inport  Port=2
  Abs1 : Abs  SaturateOnIntegerOverflow=on
  Clock1 : Clock
  Compare To Constant1 : simulink/Logic and Bit Operations/Compare To Constant  relop=>  const=0.05  OutDataTypeStr=uint8  ZeroCross=off
  Gain : Gain  Gain=-1
  Max Torque : Gain  Gain=400
  Product : Product  RndMeth=Zero
  Saturation Dynamic : simulink/Discontinuities/Saturation Dynamic  OutMin=[]  OutMax=[]  OutDataTypeStr=Inherit: Same as second input  OutDataType=sfix(16)  OutScaling=2^-10  DoSatur=off
  Torque vs speed : Lookup  InputValues=[0 1200 2000 3000 4000 5000 6000]*pi/30  Table="[400.0000  400.0000  280.0000  222.8169  179.0493  143.2394  119.3662]"
  torque : Outport
  wires:
  N rad/s/1 -> Abs1/1
  Abs1/1 -> Torque vs speed/1
  Torque/1 -> Max Torque/1
  Gain/1 -> Saturation Dynamic/3
  Max Torque/1 -> Saturation Dynamic/2
  Torque vs speed/1 -> Saturation Dynamic/1, Gain/1
  Clock1/1 -> Compare To Constant1/1
  Saturation Dynamic/1 -> Product/1
  Compare To Constant1/1 -> Product/2
  Product/1 -> torque/1

== system power_HEV_powertrain/Planetary Gear  Subsystem1/(no zero) Divide ==
  SP1 : Inport
  SP2 : Inport  Port=2
  Abs : Abs
  Abs1 : Abs
  Divide1 : Product  Inputs=*/
  Divide2 : Product  Inputs=***
  Sign : Signum
  Sign1 : Signum
  zero avoider : Saturate  UpperLimit=inf  LowerLimit=1e-12
  WR : Outport
  wires:
  SP1/1 -> Abs/1, Sign/1
  Divide2/1 -> WR/1  "Willis relation"
  SP2/1 -> Abs1/1, Sign1/1
  Abs/1 -> Divide1/1
  Abs1/1 -> zero avoider/1
  zero avoider/1 -> Divide1/2
  Divide1/1 -> Divide2/2
  Sign1/1 -> Divide2/3
  Sign/1 -> Divide2/1

== system power_HEV_powertrain/Electrical Subsystem/DC/DC Converter/Bus DC controller ==
  Ubus : Inport
  Uref : Inport  Port=2
  Current controller DISCRETE1 : Subsystem  mask(PI controller){Kp=0.001, Ki=1, Ts=Ts}
      mask prompts: Kp "Proportional gain (Kp)"; Ki "Integral gain (Ki)"; Ts "Sample time (s) :"
      mask help: Proportional-Integral Speed Controller
      mask Display: plot(0,0,100,100,[35,35,65],[70,30,30],[35,65],[45,60])
  Duty Cycles : Subsystem
  Mux : Mux  Inputs=2
  Transfer Fcn : TransferFcn  Denominator=[.0001 1]
  Unit Delay2 : UnitDelay  InitialCondition=.5  SampleTime=Ts
  Zero-Order Hold1 : ZeroOrderHold  SampleTime=Ts
  Duty cycle : Outport  InitialOutput=0
  tag scope: V_DCDC=global
  wires:
  Ubus/1 -> Zero-Order Hold1/1, Mux/2
  Uref/1 -> Current controller DISCRETE1/2(Uref), Mux/1
  Zero-Order Hold1/1 -> Transfer Fcn/1
  Unit Delay2/1 -> Duty cycle/1
  Transfer Fcn/1 -> Current controller DISCRETE1/1(UBus)
  Current controller DISCRETE1/1(Ec) -> Duty Cycles/1(Ec)
  Duty Cycles/1(dc) -> Unit Delay2/1
  Mux/1 -> [V_DCDC]

== system power_HEV_powertrain/Electrical Subsystem/DC/DC Converter/DC/DC converter ==
  Duty Cycle : Inport
  CBus : powerlib/Elements/Series RLC Branch  LConnTagsString=__new0  RConnTagsString=__new0  BranchType=RC  Resistance=0.2  Inductance=1e-3  SetiL0=off  InitialCurrent=0  Capacitance=1130e-6  Setx0=on  InitialVoltage=500  Measurements=None
  CBus1 : powerlib/Elements/Series RLC Branch  LConnTagsString=__new0  RConnTagsString=__new0  BranchType=C  Resistance=0.2  Inductance=1e-3  SetiL0=off  InitialCurrent=0  Capacitance=282e-6  Setx0=on  InitialVoltage=150  Measurements=None
  Chopper : DC6DriveInternalModels/Chopper (average model)  SnubberResistance=10e3  SnubberCapacitance=inf  Ron=1e-3  ForwardVoltages=[1.3,1.3]  IGBTParameters=[0,0]  converterType=Inverter
  L : powerlib/Elements/Series RLC Branch  LConnTagsString=__new0  RConnTagsString=__new0  BranchType=L  Resistance=0.3  Inductance=373e-6  SetiL0=off  InitialCurrent=100  Capacitance=100e-6  Setx0=off  InitialVoltage=0  Measurements=None
  Neutral2 : powerlib/Elements/Neutral  LConnTagsString=a  NodeNumber=10
  V1 : powerlib/Measurements/Voltage Measurement  PhasorSimulation=off  OutputType=Complex  PSBequivalent=0
  + : PMIOPort  Tag=PMCPort  Port=1  Side=Left
  - : PMIOPort  Tag=PMCPort  Port=2  Side=Left
  + bat. : PMIOPort  Tag=PMCPort  Port=3  Side=Right
  - bat. : PMIOPort  Tag=PMCPort  Port=4  Side=Right
  UBus : Outport
  wires:
  Duty Cycle/1 -> Chopper/1
  V1/1 -> UBus/1
  connections:
  Chopper/RConn1 -- L/RConn1
  L/LConn1 -- + bat./RConn1 -- CBus1/LConn1
  CBus1/RConn1 -- - bat./RConn1 -- Chopper/LConn2 -- -/RConn1 -- CBus/RConn1 -- V1/LConn2 -- Neutral2/LConn1
  +/RConn1 -- CBus/LConn1 -- Chopper/LConn1 -- V1/LConn1

== system power_HEV_powertrain/Electrical Subsystem/Generator Drive 30kW/Mux ==
  sig* : Inport
  m : Inport  Port=2
  Bus Creator : BusCreator  Inputs=2
  Ctrl : Outport
  wires:
  m/1 -> Bus Creator/2  "m"
  sig*/1 -> Bus Creator/1  "Signals*"
  Bus Creator/1 -> Ctrl/1
